simulink model "sim_2D_Falcon_9_traj"  (R2024b)
settings: Solver=FixedStepAuto  StartTime=0.0  StopTime=30  FixedStep=0.0001  RelTol=1e-3
settings Model: Creator=olive  LastModifiedBy=olivermcnaughton
settings DebuggingCC: UnderSpecifiedDimensionMsg=warning

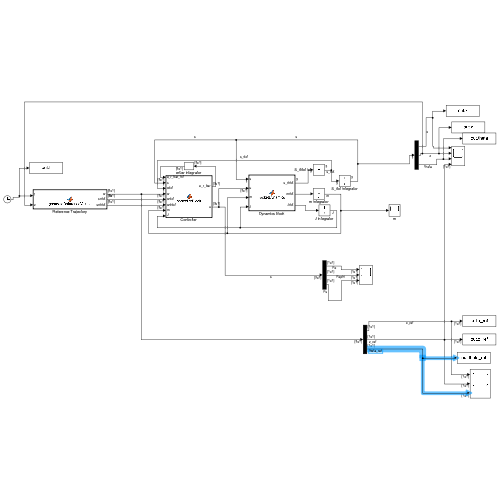
[thumbnail: Simulink's stored preview of the top-level diagram]
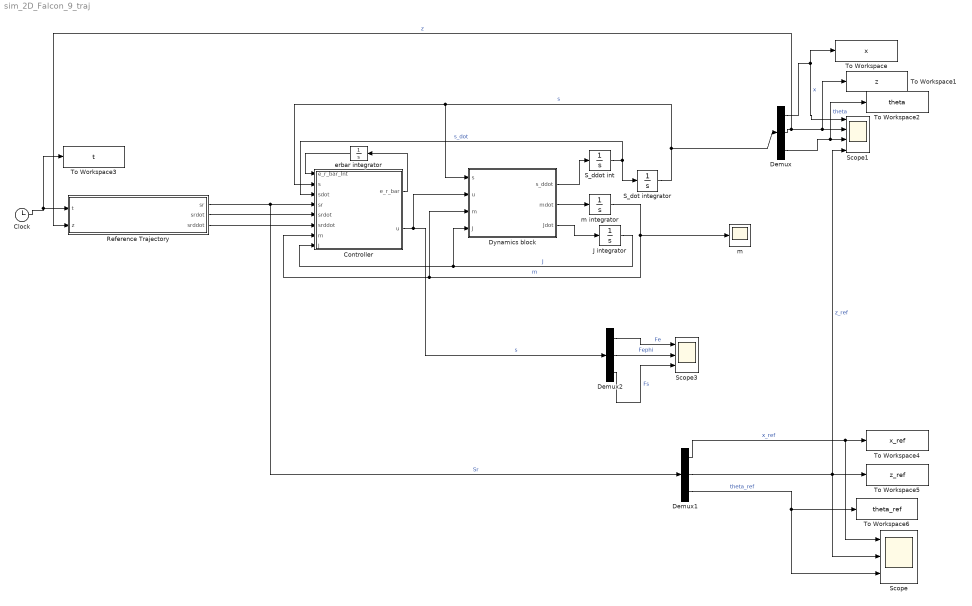
== system sim_2D_Falcon_9_traj ==
  Clock : Clock
  Controller : MATLAB Function  TreatAsAtomicUnit=on
  Demux : Demux  Outputs=3
  Demux1 : Demux  Outputs=3
  Demux2 : Demux  Outputs=3
  Dynamics block : MATLAB Function  TreatAsAtomicUnit=on
  J integrator : Integrator  InitialCondition=5
  Reference Trajectory : MATLAB Function  TreatAsAtomicUnit=on
  S_ddot int : Integrator  InitialCondition=[0; 0; 0]
  S_dot integrator : Integrator  InitialCondition=[0.3;1;0]
  Scope : Scope  NumInputPorts=3
  Scope1 : Scope  NumInputPorts=4
  Scope3 : Scope  NumInputPorts=3
  To Workspace : ToWorkspace  VariableName=x  SaveFormat=Timeseries  SampleTime=-1
  To Workspace1 : ToWorkspace  VariableName=z  SaveFormat=Timeseries  SampleTime=-1
  To Workspace2 : ToWorkspace  VariableName=theta  SaveFormat=Timeseries  SampleTime=-1
  To Workspace3 : ToWorkspace  VariableName=t  SaveFormat=Timeseries  SampleTime=-1
  To Workspace4 : ToWorkspace  VariableName=x_ref  SaveFormat=Timeseries  SampleTime=-1
  To Workspace5 : ToWorkspace  VariableName=z_ref  SaveFormat=Timeseries  SampleTime=-1
  To Workspace6 : ToWorkspace  VariableName=theta_ref  SaveFormat=Timeseries  SampleTime=-1
  erbar integrator : Integrator
  m : Scope
  m integrator : Integrator  InitialCondition=25
  wires:
  Dynamics block/1(s_ddot) -> S_ddot int/1
  Dynamics block/2(mdot) -> m integrator/1
  Dynamics block/3(Jdot) -> J integrator/1
  S_ddot int/1 -> S_dot integrator/1, Controller/3(sdot)  "s_dot"
  S_dot integrator/1 -> Dynamics block/1(s), Controller/2(s), Demux/1  "s"
  J integrator/1 -> Dynamics block/4(J), Controller/8(J)  "J"
  m integrator/1 -> Dynamics block/3(m), Controller/7(m), m/1  "m"
  Controller/1(e_r_bar) -> erbar integrator/1
  erbar integrator/1 -> Controller/1(e_r_bar_Int)
  Demux/1 -> To Workspace/1, Scope1/1  "x"
  Demux/2 -> Reference Trajectory/2(z), To Workspace1/1, Scope1/2  "z"
  Demux/3 -> To Workspace2/1, Scope1/3  "theta"
  Demux2/2 -> Scope3/2  "Fephi"
  Demux2/1 -> Scope3/1  "Fe"
  Controller/2(u) -> Demux2/1, Dynamics block/2(u)  "s"
  Demux2/3 -> Scope3/3  "Fs"
  Clock/1 -> To Workspace3/1, Reference Trajectory/1(t)
  Reference Trajectory/1(sr) -> Demux1/1, Controller/4(sr)  "Sr"
  Reference Trajectory/3(srddot) -> Controller/6(srddot)
  Reference Trajectory/2(srdot) -> Controller/5(srdot)
  Demux1/2 -> To Workspace5/1, Scope1/4, Scope/2  "z_ref"
  Demux1/1 -> Scope/1, To Workspace4/1  "x_ref"
  Demux1/3 -> To Workspace6/1, Scope/3  "theta_ref"

== matlab function sim_2D_Falcon_9_traj/Reference Trajectory ==
  data: sr output; srdot output; srddot output; t input; z input
function [sr, srdot, srddot] = generateReferenceValues(t,z)
% Generates constant reference position and velocity values for x, z, and theta
% Outputs:
%   sr: Reference position vector [x_ref; z_ref; theta_ref]
%   srdot: Reference velocity vector [x_dot_ref; z_dot_ref; theta_dot_ref]

%set position and time for each segment
%the rocket follows a trajectory of a half sine wave (middle part) then a
%semi circle for the top of the boostback portion 
%then a straight line downwards

    %End time of half sinewave
    T1 = 10;
    %End point of half sine wave
    x1 = 30;
    z1 = 40;
    
    %End time of semi circle 
    T2 = 15;
    %End point of semi circle
    x2 = 15; %gives you the position of the other side of the semi circle
    z2 = 40; %this should equal z1
    
    %Landing time of rocket
    T3 = 30;
    %Landing point of rocket
    x3 = 20; % this should be equal to x2
    z3 = 0;
    
    % Initialize reference values for safety
    x_ref = 0;
    z_ref = 0;
    theta_ref = 0;

    x_dot_ref = 0;
    z_dot_ref = 0;
    theta_dot_ref = 0;

    x_ddot_ref = 0;
    z_ddot_ref = 0;
    theta_ddot_ref = 0;

    %The first half sine wave
    if t<T1
        %reference positions
        x_ref = (-sin((pi/2) + pi*t/T1)+1)*x1/2;
        z_ref = z1*t/T1;
        theta_ref = atan(sin(pi*t/T1));
        
        %Reference Velocities
        x_dot_ref = (-pi/T1)*cos((pi/2) + pi*t/T1)*x1/2;
        z_dot_ref = z1/T1;
        theta_dot_ref = (pi/T1)*cos(pi*t/T1)/(sin(pi*t/T1)^2 + 1);

        %Reference Accelerations
        x_ddot_ref = ((pi/T1)^2)*sin((pi/2) + pi*t/T1)*x1/2;
        z_ddot_ref = 0;
        k = pi/T1;
        theta_ddot_ref = -k^2 * sin(k * t) * (3 - sin(k * t)^2) / (1 + sin(k * t)^2)^2;
    end
    %now doing the semi circle
    if t<T2 && t>=T1
        %calculate radius
        r = (x1-x2)/2; %radius 
        h = (x1+x2)/2; %x position for centre of circle
        dT = T2-T1; %Time between points
        dX = x1-x2;
        thetaMax = pi/4; %max angle at when halfway through the semi circle 
        teff = t -T1; %need to "zero" compared to the RHS of the semi circle
        %reference positions
        x_ref = h + r*cos(pi*teff/dT);
        z_ref = z1 + r*sin(pi*teff/dT);
        theta_ref = thetaMax*sin(2*pi*teff/dT + pi);
        %Reference Velocities
        x_dot_ref = (-pi/dT)*r*sin(pi*teff/dT);
        z_dot_ref = (pi/dT)*r*cos(pi*teff/dT);
        theta_dot_ref = thetaMax*(2*pi/dT)*cos(2*pi*teff/dT + pi);

        %Reference Accelerations
        x_ddot_ref = -(pi^2/dT^2)*r*cos(pi*teff/dT);
        z_ddot_ref = -(pi^2/dT^2)*r*sin(pi*teff/dT);
        theta_ddot_ref = -4*(pi^2/dT^2)*thetaMax*sin(pi*teff/dT + pi);
    end
    %now it is landing
    if t>=T2 
        % Position
        x_ref = x2; % Assuming no horizontal movement during landing
        z_ref = 1/(t^10);
        theta_ref = 0; % No rotation during landing
        
        % Velocity
        x_dot_ref = 0;
        if z<1
            z_dot_ref = 0;
            z_ref = 0;
        else
            z_dot_ref = -1;
        end
        
        theta_dot_ref = 0;
        
        % Acceleration
        x_ddot_ref = 0;
        z_ddot_ref = 0;
        theta_ddot_ref = 0;
    end
    if t>T3
        x_ref = x2;
        z_ref = 0;
        theta_ref = 0; % No rotation during landing
    end
    % Output reference values
    sr = [x_ref; z_ref; theta_ref];
    srdot = [x_dot_ref; z_dot_ref; theta_dot_ref];
    srddot = [x_ddot_ref; z_ddot_ref; theta_ddot_ref];
end

== matlab function sim_2D_Falcon_9_traj/Dynamics block ==
  data: s input size=3; u input; m input; J input; s_ddot output size=3; mdot output size=1; Jdot output size=1
function [s_ddot,mdot,Jdot] = rocketDynamics(s,u,m,J)

%initialise states
L1 = 1;
L2 = 1;
Ln = 1;
alpha1 = 0.009;
alpha2 = 0.005;
beta = 0.03;
g = 9.81;

%extract states
Fe = u(1);
Fephi = u(2);
Fs = u(3);
theta = s(3);

%find mdot and Jdot
mdot = -alpha1*(beta*Fe +abs(Fs));
Jdot = -alpha2*(beta*Fe + abs(Fs));
%update mdot and Jdot

fs = [0;-g;0];
gs = [theta/m 1/m 1/m; 1/m -theta/m -theta/m; 0 -(L1+Ln)/J L2/J]; 
s_ddot = fs + gs * u;
end

== matlab function sim_2D_Falcon_9_traj/Controller ==
  data: e_r_bar_Int input; s input; sdot input; sr input; srdot input; srddot input; m input; J input; e_r_bar output; u output
function [e_r_bar,u] = controllerBlock(e_r_bar_Int,s,sdot,sr,srdot,srddot,m,J)
% controllerBlock computes control input u for a 3-DOF system.
%
% Inputs:
%   s       = [x; z; theta] (actual position/orientation)
%   sr      = [x_r; z_r; theta_r] (reference)
%   sdot    = [xdot; zdot; thetadot] (actual velocity)
%   srdot   = [x_rdot; z_rdot; theta_rdot] (reference velocity)
%   sddot   = [xddot; zddot; thetaddot] (actual acceleration)
%   srddot  = [x_rddot; z_rddot; theta_rddot] (reference acceleration)
%
% Output:
%   u       = control input 

    % == Extract actual states ==
    x       = s(1); 
    z       = s(2);
    theta   = s(3);
    
    % == Extract reference states ==
    xr      = sr(1);
    zr      = sr(2);
    thetar  = sr(3);

    % == Extract actual velocities ==
    xdot    = sdot(1);
    zdot    = sdot(2);
    thetadot= sdot(3);

    % == Extract reference velocities ==
    xrdot   = srdot(1);
    zrdot   = srdot(2);
    thetardot = srdot(3);

    % == Constants / Gains (fill in correct values!) ==
    g       = 9.81;     % Gravity
    L1      = 1;      % etc... fill in or remove as needed
    L2      = 1;
    Ln      = 1;
    kx      = 5;        % Gains for position errors
    kz      = 6;
    ktheta  = 5;
    
    % define f_s
    f_s = [0; -g; 0];  
   
    % Define gs
    g_s = [ theta/m   1/m   1/m;
            1/m    -theta/m  -theta/m;
            0     -(L1+Ln)/J     L2/J ];
        
    % Gains for the error feedback
    K_s = diag([0.5, 0.1, 0.25]);
    K_i = diag([0.25, 0.0, 0.25]);  
    K_r = diag([kx, kz, ktheta]);   
    
    % == Errors ==
    % Position error:
    e_pos  = [x - xr; z - zr; theta - thetar];
    
    % Velocity error:
    e_vel  = [xdot - xrdot; zdot - zrdot; thetadot - thetardot];  

    % == Now compute your feedforward and feedback terms ==
    f_s_bar = f_s - srddot + K_r * e_vel; 
  

    e_r_bar = e_vel + K_r * e_pos;  

    % == Calculate u 
    u = g_s\( -f_s_bar - K_s * e_r_bar - K_i * e_r_bar_Int );
    
    %set bounds for u 
    u(1) =  max(0, min(6486, u(1)));  %We need to bound Fe min = 0N max = 6486N
    u(2) =  max(-1678.7, min(1678.7, u(2)));  %Need to Bound Fephi 
    u(3) =  max(-130, min(130, u(3)));  %Need to bound Fs

end
